simulink model "simulRMPC"  (R2017a)
settings: Solver=VariableStepAuto  StartTime=0.0  StopTime=tSimulacion  RelTol=1e-3
values from neighbouring files (symbols this model uses):
  Acont = [0 1;0 0]    [delayRMPC.m]    (also in runPL.m; runRMPC.m; simul1.mat = [0  1; 0  0]; simul10.mat = [0  1; 0  0])
  Ades = [rell1,ALB;rell1,AUB;rell2,ADeltaLB,rell3;rell2,rell3,ADeltaLB;rell2,ADeltaUB,rell3;rell2,rell3,ADeltaUB]    [defRestricciones.m]    (also in simul1.mat = [0 0 0 0 0 0 0 0 0 0 0 0 ... (1080 elements, 36x30)]; simul10.mat = [0 0 0 0 0 0 0 0 0 0 0 0 ... (1080 elements, 36x30)]; simul11.mat = [0 0 0 0 0 0 0 0 0 0 0 0 ... (1080 elements, 36x30)]; simul12.mat = [0 0 0 0 0 0 0 0 0 0 0 0 ... (1080 elements, 36x30)])
  Bcont = [0;1]    [delayRMPC.m]    (also in runPL.m; runRMPC.m; simul1.mat = [0 1]; simul10.mat = [0 1])
  bdes = [bLB;bUB;bDeltaLB;bDeltaUB]    [defRestricciones.m]    (also in simul1.mat = [1.5 1.5 1.5 1.5 1.5 1.5 1.5 1.5 1.5 1.5 1 1 ... (36 element; simul10.mat = [1.5 1.5 1.5 1.5 1.5 1.5 1.5 1.5 1.5 1.5 1 1 ... (36 element; simul11.mat = [1.5 1.5 1.5 1.5 1.5 1.5 1.5 1.5 1.5 1.5 1 1 ... (36 element; simul12.mat = [1.5 1.5 1.5 1.5 1.5 1.5 1.5 1.5 1.5 1.5 1 1 ... (36 element)
  Ccont = eye(2)    [delayRMPC.m]    (also in runPL.m; runRMPC.m; simul1.mat = [1  0; 0  1]; simul10.mat = [1  0; 0  1])
  d = 2    [delayRMPC.m]    (also in runPL.m; runRMPC.m; simul1.mat; simul10.mat)
  Dcont = [0;0]    [delayRMPC.m]    (also in runPL.m; runRMPC.m; simul1.mat = [0 0]; simul10.mat = [0 0])
  Ldes = input('Valor de spacing deseado (m): ')    [delayRMPC.m]    (also in runPL.m; runRMPC.m = 2; simul1.mat = 2; simul10.mat = 2)
  meanError = -0.0091    [delayRMPC.m]    (also in runPL.m; runRMPC.m; simul1.mat = 0.0164; simul10.mat = 0.0164)
  MError =     [simul1.mat]    (also in simul10.mat; simul11.mat; simul12.mat; simul13.mat)
  nPasos = (length(bdes)+4)/8    [comprimirRestricciones.m]    (also in delayRMPC.m = input('Numero de pasos prediccion: '); runPL.m = input('Numero de pasos prediccion: '); runRMPC.m = 4; simul1.mat = 5)
  ts = input('Tiempo de muestreo (s): ')    [delayRMPC.m]    (also in runPL.m; runRMPC.m = 0.1; simul1.mat = 0.4; simul10.mat = 0.5)
  v0Bici1 = 1    [delayRMPC.m]    (also in runPL.m; runRMPC.m; simul1.mat; simul10.mat)
  v0Leader = input('Velocidad lider (m/s)(2.7,4.16,5)')    [delayRMPC.m]    (also in runPL.m; runRMPC.m = 2.7; simul1.mat = 2.7; simul10.mat = 2.7)
  varError = varError^2    (= 0.15800625)    [delayRMPC.m]    (also in runPL.m; runRMPC.m; simul1.mat = 0.14661241; simul10.mat = 0.14661241)
  x0Bici1 = -10    [delayRMPC.m]    (also in runPL.m; runRMPC.m; simul1.mat; simul10.mat)
  x0Leader = 0    [delayRMPC.m]    (also in runPL.m; runRMPC.m; simul1.mat; simul10.mat)
undefined symbols (not defined in the file or in its folder): solveRMPC
settings Model: Creator=tlara  LastModifiedBy=tlara

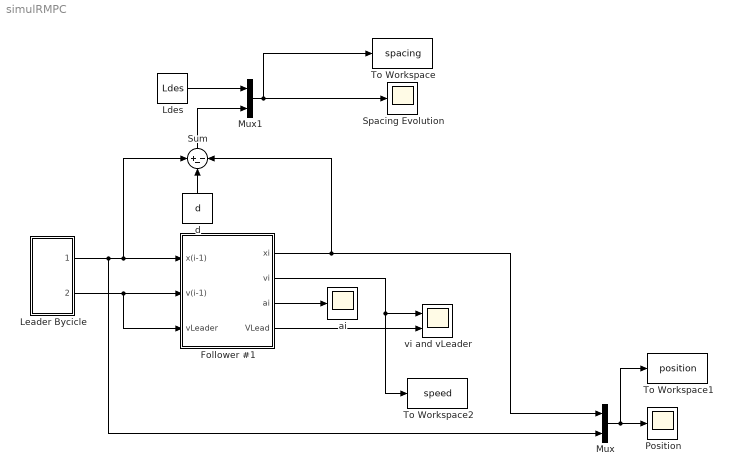
== system simulRMPC ==
  "Follower #1 " : Subsystem
  Ldes : Constant  Value=Ldes
  "Leader Bycicle " : Subsystem
  Mux : Mux  Inputs=2
  Mux1 : Mux  Inputs=2
  Position : Scope
  Spacing Evolution : Scope
  Sum : Sum  Inputs=+--
  To Workspace : ToWorkspace  VariableName=spacing  SaveFormat=Timeseries  SampleTime=-1
  To Workspace1 : ToWorkspace  VariableName=position  SaveFormat=Timeseries  SampleTime=-1
  To Workspace2 : ToWorkspace  VariableName=speed  SaveFormat=Timeseries  SampleTime=-1
  ai : Scope
  "d " : Constant  Value=d
  vi and vLeader : Scope  NumInputPorts=2
  wires:
  "Leader Bycicle "/2(Speed) -> "Follower #1 "/3(vLeader), "Follower #1 "/2(v(i-1))
  Mux1/1 -> To Workspace/1, Spacing Evolution/1
  Ldes/1 -> Mux1/1
  "d "/1 -> Sum/2
  Sum/1 -> Mux1/2
  Mux/1 -> To Workspace1/1, Position/1
  "Follower #1 "/1(xi) -> Mux/1, Sum/3
  "Leader Bycicle "/1(Position) -> "Follower #1 "/1(x(i-1)), Sum/1, Mux/2
  "Follower #1 "/3(ai) -> ai/1
  "Follower #1 "/4(VLead) -> vi and vLeader/2
  "Follower #1 "/2(vi) -> To Workspace2/1, vi and vLeader/1

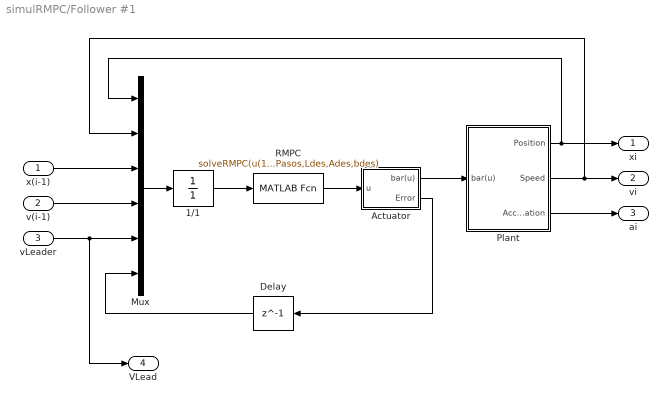
== system simulRMPC/Follower #1  ==
  x(i-1) : Inport
  v(i-1) : Inport  Port=2
  vLeader : Inport  Port=3
  "1/1 " : DiscreteTransferFcn  Denominator=[1]  SampleTime=ts
  Actuator : Subsystem
  Delay : Delay  DelayLength=1  InitialCondition=0  SampleTime=ts
  Mux : Mux  Inputs=6
  Plant : Subsystem
  RMPC : MATLABFcn  MATLABFcn=solveRMPC(u(1),u(2),u(3),u(4),u(5),u(6),MError,nPasos,Ldes,Ades,bdes)  OutputDimensions=1  OutputSignalType=real
  xi : Outport
  vi : Outport  Port=2
  ai : Outport  Port=3
  VLead : Outport  Port=4
  wires:
  vLeader/1 -> VLead/1, Mux/5
  v(i-1)/1 -> Mux/4
  x(i-1)/1 -> Mux/3
  Mux/1 -> "1/1 "/1
  "1/1 "/1 -> RMPC/1
  RMPC/1 -> Actuator/1(u)
  Actuator/1(bar(u)) -> Plant/1(bar(u))
  Plant/1(Position) -> Mux/1, xi/1
  Plant/2("Speed ") -> Mux/2, vi/1
  Plant/3(Acceleration) -> ai/1
  Actuator/2(Error) -> Delay/1
  Delay/1 -> Mux/6

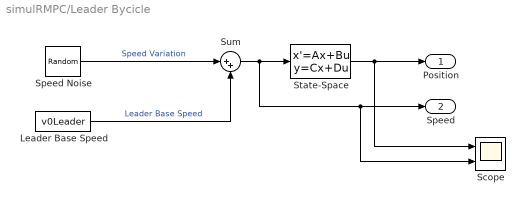
== system simulRMPC/Leader Bycicle  ==
  "Leader Base Speed " : Constant  Value=v0Leader
  Scope : Scope  NumInputPorts=2
  Speed Noise : RandomNumber  Variance=0.02  SampleTime=ts
  State-Space : StateSpace  A=[0]  B=[1]  C=[1]  D=[0]  X0=[x0Leader]  ContinuousStateAttributes='position'
  Sum : Sum  Inputs=|++
  Position : Outport
  Speed : Outport  Port=2
  wires:
  "Leader Base Speed "/1 -> Sum/2  "Leader Base Speed"
  Speed Noise/1 -> Sum/1  "Speed Variation"
  State-Space/1 -> Position/1, Scope/1
  Sum/1 -> State-Space/1, Speed/1, Scope/2

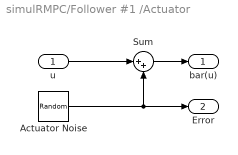
== system simulRMPC/Follower #1 /Actuator ==
  u : Inport
  Actuator Noise : RandomNumber  Mean=meanError  Variance=varError  SampleTime=ts
  Sum : Sum  Inputs=|++
  bar(u) : Outport
  Error : Outport  Port=2
  wires:
  Sum/1 -> bar(u)/1
  u/1 -> Sum/1
  Actuator Noise/1 -> Sum/2, Error/1

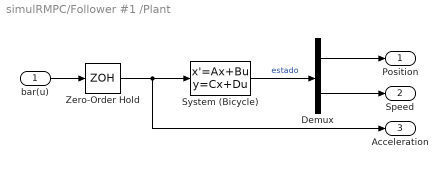
== system simulRMPC/Follower #1 /Plant ==
  bar(u) : Inport
  Demux : Demux  Outputs=2
  "System (Bicycle) " : StateSpace  A=Acont  B=Bcont  C=Ccont  D=Dcont  X0=[x0Bici1,v0Bici1]  ContinuousStateAttributes='Position'
  Zero-Order Hold : ZeroOrderHold  SampleTime=ts
  Position : Outport
  "Speed " : Outport  Port=2
  Acceleration : Outport  Port=3
  wires:
  bar(u)/1 -> Zero-Order Hold/1
  Zero-Order Hold/1 -> Acceleration/1, "System (Bicycle) "/1
  Demux/1 -> Position/1
  "System (Bicycle) "/1 -> Demux/1  "estado"
  Demux/2 -> "Speed "/1
